simulink model "controladorContinua"  (R2021a)
settings: Solver=ode45  StartTime=0.0  StopTime=60  RelTol=1e-3
values from neighbouring files (symbols this model uses):
  AL = double(subs(A_par))    [1modeloMATEMATICOFINAL.m]    (also in modeloMATEMATICOFINAL.m)
  BL = double(subs(B_par))    [1modeloMATEMATICOFINAL.m]    (also in modeloMATEMATICOFINAL.m)
  Blo = 8.18575752786119e-06    (= 8.18575752786e-06)    [1modeloMATEMATICOFINAL.m]    (also in modeloMATEMATICOFINAL.m)
  Bmo = 2.02156082362446e-07    (= 2.02156082362e-07)    [1modeloMATEMATICOFINAL.m]    (also in modeloMATEMATICOFINAL.m)
  CL = double(subs(C_par))    [1modeloMATEMATICOFINAL.m]    (also in modeloMATEMATICOFINAL.m = [0 1 0)
  DL = double(subs(D_par))    [1modeloMATEMATICOFINAL.m]    (also in modeloMATEMATICOFINAL.m = [0)
  do = 0.06862-0.021    (= 0.04762)    [1modeloMATEMATICOFINAL.m]    (also in modeloMATEMATICOFINAL.m)
  go = 9.81    [1modeloMATEMATICOFINAL.m]    (also in modeloMATEMATICOFINAL.m)
  Jlo = 0.00100697016255642    (= 0.00100697016256)    [1modeloMATEMATICOFINAL.m]    (also in modeloMATEMATICOFINAL.m)
  Jmo = 2.08549279330578e-07    (= 2.08549279331e-07)    [1modeloMATEMATICOFINAL.m]    (also in modeloMATEMATICOFINAL.m)
  Kes = K(:,1:n)    [1modeloMATEMATICOFINAL.m]
  Ki = -K(:,n+1:end)    [1modeloMATEMATICOFINAL.m]    (also in modeloMATEMATICOFINAL.m = 3.82295123971)
  Kio = 0.00119530882984502    (= 0.00119530882985)    [1modeloMATEMATICOFINAL.m]    (also in modeloMATEMATICOFINAL.m)
  Kvo = 0.0035694528924319    (= 0.00356945289243)    [1modeloMATEMATICOFINAL.m]    (also in modeloMATEMATICOFINAL.m)
  Lo = 0.667669785204658    (= 0.667669785205)    [1modeloMATEMATICOFINAL.m]    (also in modeloMATEMATICOFINAL.m)
  mo = 0.17244    [1modeloMATEMATICOFINAL.m]    (also in modeloMATEMATICOFINAL.m)
  no = 120    [1modeloMATEMATICOFINAL.m]    (also in modeloMATEMATICOFINAL.m)
  Ro = 5.15610211779038    (= 5.15610211779)    [1modeloMATEMATICOFINAL.m]    (also in modeloMATEMATICOFINAL.m)
  Tm = 0.03    [1modeloMATEMATICOFINAL.m]    (also in modeloMATEMATICOFINAL.m)
  Vin0 = Ro*X10    (= 0)    [1modeloMATEMATICOFINAL.m]    (also in modeloMATEMATICOFINAL.m)
  X10 = 0    [1modeloMATEMATICOFINAL.m]    (also in modeloMATEMATICOFINAL.m)
  X20 = 0    [1modeloMATEMATICOFINAL.m]    (also in modeloMATEMATICOFINAL.m)
  X30 = 0    [1modeloMATEMATICOFINAL.m]    (also in modeloMATEMATICOFINAL.m)
libraries: cstblocks x12
settings Model: Creator=hubertdelgado  LastModifiedBy=hubertdelgado

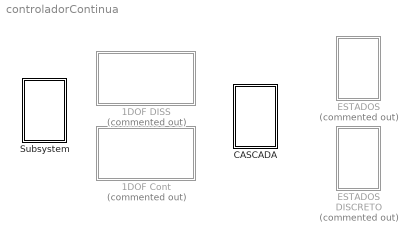
== system controladorContinua ==
  1DOF Cont : Subsystem  Commented=on
  1DOF DISS : Subsystem  Commented=on
  CASCADA : Subsystem
  ESTADOS : Subsystem  Commented=on
  ESTADOS DISCRETO : Subsystem  Commented=on
  Subsystem : Subsystem

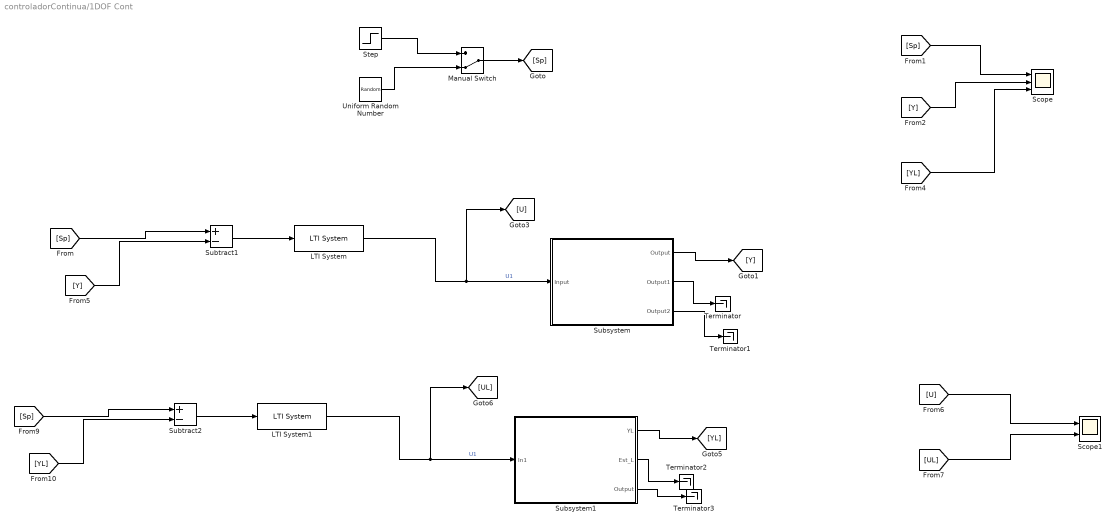
== system controladorContinua/1DOF Cont ==
  LTI System : cstblocks/LTI System  sys=Cpids  IC=[]
  LTI System1 : cstblocks/LTI System  sys=Cpids  IC=[]
  Manual Switch : ManualSwitch  CurrentSetting=0
  Scope : Scope  NumInputPorts=3
  Scope1 : Scope  NumInputPorts=2
  Step : Step  Time=0  After=0  SampleTime=0
  Subsystem : Subsystem
  Subsystem1 : Subsystem
  Subtract1 : Sum  Inputs=+-
  Subtract2 : Sum  Inputs=+-
  Terminator{,1..3} (4 alike) : Terminator
  Uniform Random Number : UniformRandomNumber  Minimum=-40*(pi/180)  Maximum=40*(pi/180)  SampleTime=8
  wires:
  Manual Switch/1 -> [Sp]
  Uniform Random Number/1 -> Manual Switch/2
  [U] -> Scope1/1
  [UL] -> Scope1/2
  Step/1 -> Manual Switch/1
  Subtract1/1 -> LTI System/1
  LTI System/1 -> Subsystem/1(Input), [U]  "U1"
  [Sp] -> Subtract1/1
  [Y] -> Subtract1/2
  Subsystem/1(Output) -> [Y]
  Subtract2/1 -> LTI System1/1
  [YL] -> Subtract2/2
  LTI System1/1 -> Subsystem1/1(In1), [UL]  "U1"
  Subsystem1/2(Est_L) -> Terminator2/1
  Subsystem1/1(YL) -> [YL]
  [Sp] -> Subtract2/1
  [Sp] -> Scope/1
  [Y] -> Scope/2
  [YL] -> Scope/3
  Subsystem/2(Output1) -> Terminator/1
  Subsystem/3(Output2) -> Terminator1/1
  Subsystem1/3(Output) -> Terminator3/1

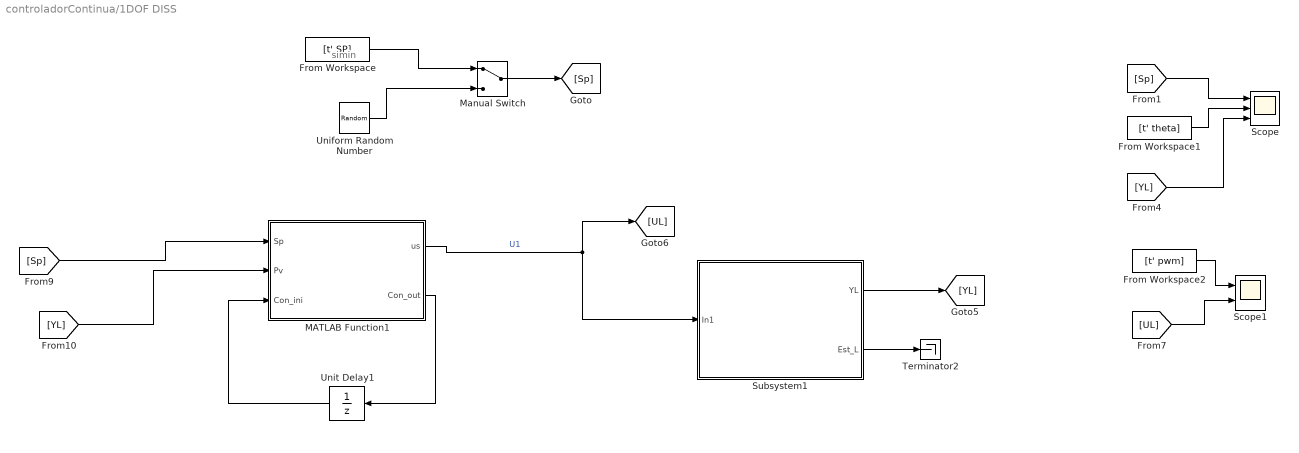
== system controladorContinua/1DOF DISS ==
  note: simin
  From Workspace : FromWorkspace  VariableName=[t' SP]
  From Workspace1 : FromWorkspace  VariableName=[t' theta]
  From Workspace2 : FromWorkspace  VariableName=[t' pwm]
  MATLAB Function1 : MATLAB Function  TreatAsAtomicUnit=on
  Manual Switch : ManualSwitch
  Scope : Scope  NumInputPorts=3
  Scope1 : Scope  NumInputPorts=2
  Subsystem1 : Subsystem
  Terminator2 : Terminator
  Uniform Random Number : UniformRandomNumber  Minimum=-40*(pi/180)  Maximum=40*(pi/180)  SampleTime=8
  Unit Delay1 : UnitDelay  InitialCondition=zeros(4,1)  SampleTime=Tm  HasFrameUpgradeWarning=on
  wires:
  Manual Switch/1 -> [Sp]
  Uniform Random Number/1 -> Manual Switch/2
  From Workspace2/1 -> Scope1/1
  [UL] -> Scope1/2
  From Workspace/1 -> Manual Switch/1
  [YL] -> MATLAB Function1/2(Pv)
  MATLAB Function1/1(us) -> Subsystem1/1(In1), [UL]  "U1"
  Subsystem1/2(Est_L) -> Terminator2/1
  Subsystem1/1(YL) -> [YL]
  [Sp] -> Scope/1
  From Workspace1/1 -> Scope/2
  [YL] -> Scope/3
  Unit Delay1/1 -> MATLAB Function1/3(Con_ini)
  [Sp] -> MATLAB Function1/1(Sp)
  MATLAB Function1/2(Con_out) -> Unit Delay1/1

== system controladorContinua/CASCADA ==
  LTI System : cstblocks/LTI System  sys=C11  IC=[]
  LTI System1 : cstblocks/LTI System  sys=G11  IC=[]
  LTI System2 : cstblocks/LTI System  sys=G21  IC=[]
  LTI System3 : cstblocks/LTI System  sys=C21  IC=[]
  MATLAB Function1 : MATLAB Function  Commented=on  TreatAsAtomicUnit=on
  Scope : Scope  NumInputPorts=2
  Scope1 : Scope  Commented=on  NumInputPorts=2
  Scope3 : Scope  Commented=on
  Subsystem1 : Subsystem  Commented=on
  Subtract : Sum  Inputs=+-
  Subtract1 : Sum  Inputs=+-
  Uniform Random Number : UniformRandomNumber  Minimum=-65*(pi/180)  Maximum=65*(pi/180)  SampleTime=8
  Unit Delay1 : UnitDelay  Commented=on  InitialCondition=zeros(8,1)  SampleTime=Tm  HasFrameUpgradeWarning=on
  wires:
  MATLAB Function1/1(u2) -> Subsystem1/1(In1), Scope3/1
  MATLAB Function1/2(Con_out) -> Unit Delay1/1
  Unit Delay1/1 -> MATLAB Function1/4(Con_ini)
  Subsystem1/1(YL) -> Scope1/2, MATLAB Function1/2(Pv)  "Pv"
  Subtract/1 -> LTI System/1  "Pv1"
  Subtract1/1 -> LTI System3/1
  LTI System2/1 -> Scope/1, Subtract1/2  "Pv"
  Uniform Random Number/1 -> Scope1/1, MATLAB Function1/1(Sp), Scope/2, Subtract1/1  "Sp"
  LTI System3/1 -> Subtract/1  "Sp1"
  LTI System/1 -> LTI System1/1
  Subsystem1/2(WL) -> MATLAB Function1/3(Pv1)
  LTI System1/1 -> Subtract/2, LTI System2/1

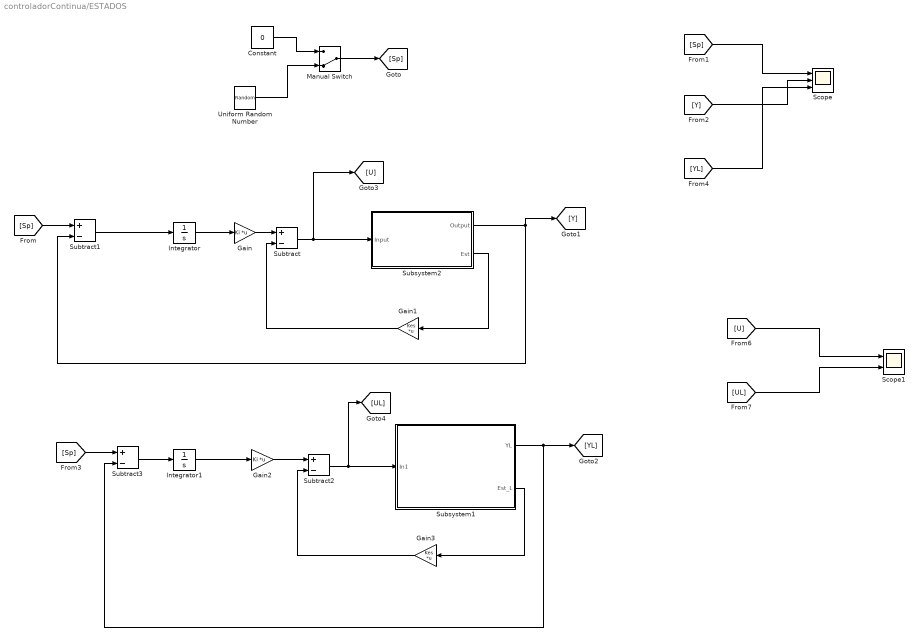
== system controladorContinua/ESTADOS ==
  Constant : Constant  Value=0
  Gain : Gain  Gain=Ki  Multiplication=Matrix(K*u)
  Gain1 : Gain  Gain=Kes  Multiplication=Matrix(K*u)
  Gain2 : Gain  Gain=Ki  Multiplication=Matrix(K*u)
  Gain3 : Gain  Gain=Kes  Multiplication=Matrix(K*u)
  Integrator : Integrator
  Integrator1 : Integrator
  Manual Switch : ManualSwitch  CurrentSetting=0
  Scope : Scope  NumInputPorts=3
  Scope1 : Scope  NumInputPorts=2
  Subsystem1 : Subsystem
  Subsystem2 : Subsystem
  Subtract{,1..3} (4 alike) : Sum  Inputs=+-
  Uniform Random Number : UniformRandomNumber  Minimum=-70*(pi/180)  Maximum=70*(pi/180)  SampleTime=8
  wires:
  Subsystem2/1(Output) -> Subtract1/2, [Y]
  Constant/1 -> Manual Switch/1
  Subsystem2/2(Est) -> Gain1/1
  Subtract/1 -> Subsystem2/1(Input), [U]
  Gain1/1 -> Subtract/2
  [YL] -> Scope/3
  Subtract2/1 -> [UL], Subsystem1/1(In1)
  Manual Switch/1 -> [Sp]
  Gain/1 -> Subtract/1
  [Sp] -> Subtract1/1
  [Sp] -> Subtract3/1
  Gain2/1 -> Subtract2/1
  Subsystem1/1(YL) -> [YL], Subtract3/2
  Subsystem1/2(Est_L) -> Gain3/1
  Gain3/1 -> Subtract2/2
  Integrator/1 -> Gain/1
  Subtract1/1 -> Integrator/1
  Integrator1/1 -> Gain2/1
  Subtract3/1 -> Integrator1/1
  Uniform Random Number/1 -> Manual Switch/2
  [Y] -> Scope/2
  [Sp] -> Scope/1
  [U] -> Scope1/1
  [UL] -> Scope1/2

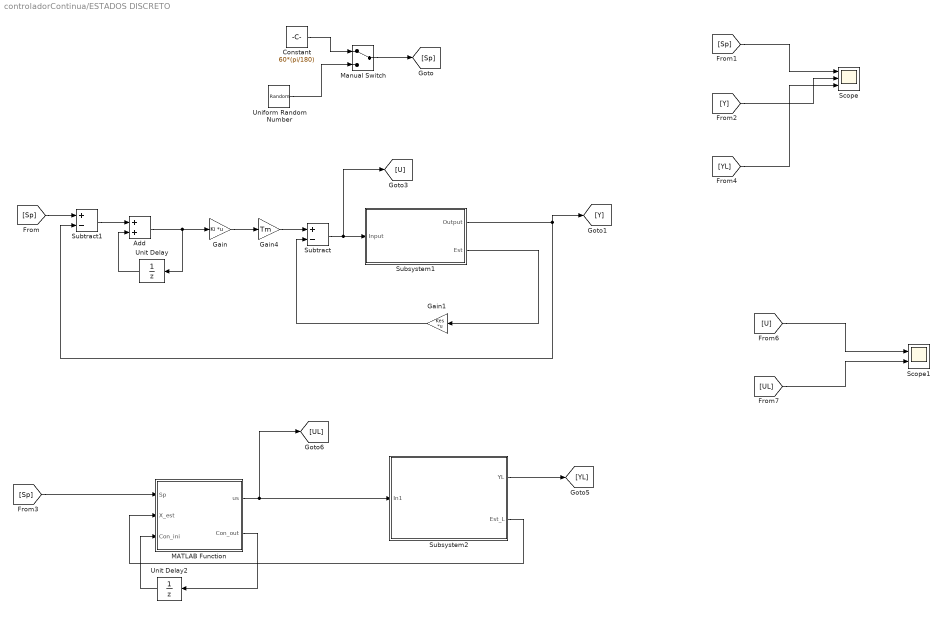
== system controladorContinua/ESTADOS DISCRETO ==
  Add : Sum
  Constant : Constant  Value=60*(pi/180)
  Gain : Gain  Gain=Ki  Multiplication=Matrix(K*u)
  Gain1 : Gain  Gain=Kes  Multiplication=Matrix(K*u)
  Gain4 : Gain  Gain=Tm
  MATLAB Function : MATLAB Function  TreatAsAtomicUnit=on
  Manual Switch : ManualSwitch
  Scope : Scope  NumInputPorts=3
  Scope1 : Scope  NumInputPorts=2
  Subsystem1 : Subsystem
  Subsystem2 : Subsystem
  Subtract : Sum  Inputs=+-
  Subtract1 : Sum  Inputs=+-
  Uniform Random Number : UniformRandomNumber  Minimum=-60*(pi/180)  Maximum=60*(pi/180)  SampleTime=8
  Unit Delay : UnitDelay  SampleTime=Tm  HasFrameUpgradeWarning=on
  Unit Delay2 : UnitDelay  InitialCondition=zeros(1,2)  SampleTime=Tm  HasFrameUpgradeWarning=on
  wires:
  Subsystem1/1(Output) -> [Y], Subtract1/2
  Subsystem1/2(Est) -> Gain1/1
  Subtract/1 -> Subsystem1/1(Input), [U]
  Gain1/1 -> Subtract/2
  [Sp] -> Subtract1/1
  Subtract1/1 -> Add/1
  Unit Delay/1 -> Add/2
  Add/1 -> Gain/1, Unit Delay/1
  Gain/1 -> Gain4/1
  Gain4/1 -> Subtract/1
  MATLAB Function/1(us) -> Subsystem2/1(In1), [UL]
  [Sp] -> MATLAB Function/1(Sp)
  MATLAB Function/2(Con_out) -> Unit Delay2/1
  Unit Delay2/1 -> MATLAB Function/3(Con_ini)
  Uniform Random Number/1 -> Manual Switch/2
  [Y] -> Scope/2
  [Sp] -> Scope/1
  [UL] -> Scope1/2
  [U] -> Scope1/1
  [YL] -> Scope/3
  Manual Switch/1 -> [Sp]
  Constant/1 -> Manual Switch/1
  Subsystem2/2(Est_L) -> MATLAB Function/2(X_est)
  Subsystem2/1(YL) -> [YL]

== system controladorContinua/Subsystem ==
  1 DOF CONTINUA : Subsystem  Commented=on
  1DOF DISCRETA : Subsystem  Commented=on
  2 DOF CONTINUA : Subsystem  Commented=on
  2 DOF DISCRETA : Subsystem  Commented=on

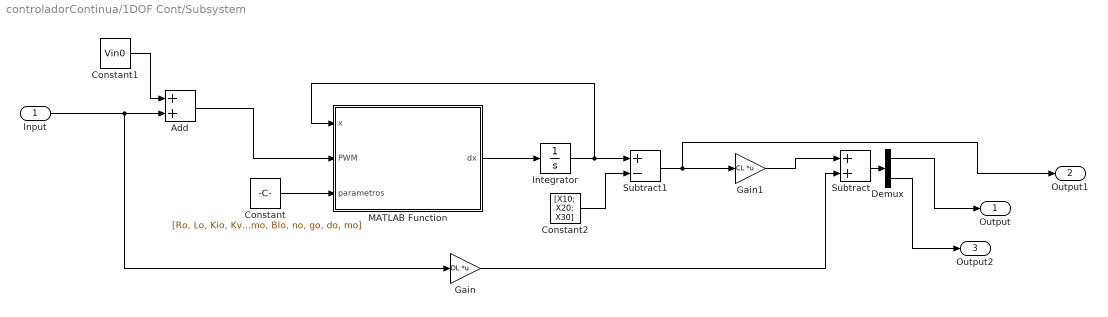
== system controladorContinua/1DOF Cont/Subsystem ==
  Input : Inport
  Add : Sum
  Constant : Constant  Value=[Ro, Lo, Kio, Kvo, Jmo, Jlo, Bmo, Blo, no, go, do, mo]
  Constant1 : Constant  Value=Vin0
  Constant2 : Constant  Value=[X10; X20; X30]
  Demux : Demux  Outputs=2
  Gain : Gain  Gain=DL  Multiplication=Matrix(K*u)
  Gain1 : Gain  Gain=CL  Multiplication=Matrix(K*u)
  Integrator : Integrator  InitialCondition=[X10; X20; X30]
  MATLAB Function : MATLAB Function  TreatAsAtomicUnit=on
  Subtract : Sum
  Subtract1 : Sum  Inputs=+-
  Output : Outport
  Output1 : Outport  Port=2
  Output2 : Outport  Port=3
  wires:
  Integrator/1 -> Subtract1/1, MATLAB Function/1(x)
  Add/1 -> MATLAB Function/2(PWM)
  Subtract1/1 -> Output1/1, Gain1/1
  MATLAB Function/1(dx) -> Integrator/1
  Constant1/1 -> Add/1
  Constant2/1 -> Subtract1/2
  Constant/1 -> MATLAB Function/3(parametros)
  Gain1/1 -> Subtract/1
  Gain/1 -> Subtract/2
  Input/1 -> Gain/1, Add/2
  Subtract/1 -> Demux/1
  Demux/1 -> Output/1
  Demux/2 -> Output2/1

== system controladorContinua/1DOF Cont/Subsystem1 ==
  In1 : Inport
  Add : Sum
  Add1 : Sum
  Demux : Demux  Outputs=2
  Gain : Gain  Gain=CL  Multiplication=Matrix(K*u)
  Gain1 : Gain  Gain=AL  Multiplication=Matrix(K*u)
  Gain2 : Gain  Gain=DL  Multiplication=Matrix(K*u)
  Gain3 : Gain  Gain=BL  Multiplication=Matrix(K*u)
  Integrator : Integrator
  YL : Outport
  Est_L : Outport  Port=2
  Output : Outport  Port=3
  wires:
  Gain/1 -> Add/2
  Integrator/1 -> Gain/1, Est_L/1, Gain1/1
  Add1/1 -> Integrator/1
  Gain1/1 -> Add1/2
  Gain2/1 -> Add/1
  Gain3/1 -> Add1/1
  In1/1 -> Gain2/1, Gain3/1
  Add/1 -> Demux/1
  Demux/1 -> YL/1
  Demux/2 -> Output/1

== system controladorContinua/1DOF DISS/Subsystem1 ==
  In1 : Inport
  Add : Sum
  Add1 : Sum
  Gain : Gain  Gain=CL  Multiplication=Matrix(K*u)
  Gain1 : Gain  Gain=AL  Multiplication=Matrix(K*u)
  Gain2 : Gain  Gain=DL  Multiplication=Matrix(K*u)
  Gain3 : Gain  Gain=BL  Multiplication=Matrix(K*u)
  Integrator : Integrator
  YL : Outport
  Est_L : Outport  Port=2
  wires:
  Gain/1 -> Add/2
  Integrator/1 -> Gain/1, Est_L/1, Gain1/1
  Add1/1 -> Integrator/1
  Gain1/1 -> Add1/2
  Gain2/1 -> Add/1
  Gain3/1 -> Add1/1
  Add/1 -> YL/1
  In1/1 -> Gain2/1, Gain3/1

== system controladorContinua/CASCADA/Subsystem1 ==
  In1 : Inport
  Add : Sum
  Add1 : Sum
  Demux : Demux  Outputs=2
  Gain : Gain  Gain=CL  Multiplication=Matrix(K*u)
  Gain1 : Gain  Gain=AL  Multiplication=Matrix(K*u)
  Gain2 : Gain  Gain=DL  Multiplication=Matrix(K*u)
  Gain3 : Gain  Gain=BL  Multiplication=Matrix(K*u)
  Integrator : Integrator
  YL : Outport
  WL : Outport  Port=2
  wires:
  Gain/1 -> Add/2
  Integrator/1 -> Gain/1, Gain1/1
  Add1/1 -> Integrator/1
  Gain1/1 -> Add1/2
  Gain2/1 -> Add/1
  Gain3/1 -> Add1/1
  In1/1 -> Gain2/1, Gain3/1
  Add/1 -> Demux/1
  Demux/1 -> YL/1
  Demux/2 -> WL/1

== system controladorContinua/ESTADOS/Subsystem1 ==
  In1 : Inport
  Add : Sum
  Add1 : Sum
  Gain : Gain  Gain=CL  Multiplication=Matrix(K*u)
  Gain1 : Gain  Gain=AL  Multiplication=Matrix(K*u)
  Gain2 : Gain  Gain=DL  Multiplication=Matrix(K*u)
  Gain3 : Gain  Gain=BL  Multiplication=Matrix(K*u)
  Integrator : Integrator
  YL : Outport
  Est_L : Outport  Port=2
  wires:
  Gain/1 -> Add/2
  Integrator/1 -> Gain/1, Est_L/1, Gain1/1
  Add1/1 -> Integrator/1
  Gain1/1 -> Add1/2
  Gain2/1 -> Add/1
  Gain3/1 -> Add1/1
  Add/1 -> YL/1
  In1/1 -> Gain2/1, Gain3/1

== system controladorContinua/ESTADOS/Subsystem2 ==
  Input : Inport
  Add : Sum
  Constant : Constant  Value=[Ro,Lo,Kio, Kvo, Jmo, Jlo, Bmo, Blo, no, go, do, mo]
  Constant1 : Constant  Value=Vin0
  Constant2 : Constant  Value=[X10; X20]
  Gain1 : Gain  Gain=CL  Multiplication=Matrix(K*u)
  Integrator : Integrator  InitialCondition=[X10; X20]
  MATLAB Function : MATLAB Function  TreatAsAtomicUnit=on
  Subtract1 : Sum  Inputs=+-
  Output : Outport
  Est : Outport  Port=2
  wires:
  Add/1 -> MATLAB Function/2(PWM)
  Constant2/1 -> Subtract1/2
  Constant1/1 -> Add/1
  Input/1 -> Add/2
  MATLAB Function/1(dx) -> Integrator/1
  Constant/1 -> MATLAB Function/3(parametros)
  Integrator/1 -> Subtract1/1, MATLAB Function/1(x)
  Subtract1/1 -> Est/1, Gain1/1
  Gain1/1 -> Output/1

== system controladorContinua/ESTADOS DISCRETO/Subsystem1 ==
  Input : Inport
  Add : Sum
  Constant : Constant  Value=[Ro,Lo,Kio, Kvo, Jmo, Jlo, Bmo, Blo, no, go, do, mo]
  Constant1 : Constant  Value=Vin0
  Constant2 : Constant  Value=[X10; X20]
  Gain1 : Gain  Gain=CL  Multiplication=Matrix(K*u)
  Integrator : Integrator  InitialCondition=[X10; X20]
  MATLAB Function : MATLAB Function  TreatAsAtomicUnit=on
  Subtract1 : Sum  Inputs=+-
  Output : Outport
  Est : Outport  Port=2
  wires:
  Add/1 -> MATLAB Function/2(PWM)
  Constant2/1 -> Subtract1/2
  Constant1/1 -> Add/1
  Input/1 -> Add/2
  MATLAB Function/1(dx) -> Integrator/1
  Constant/1 -> MATLAB Function/3(parametros)
  Integrator/1 -> Subtract1/1, MATLAB Function/1(x)
  Subtract1/1 -> Est/1, Gain1/1
  Gain1/1 -> Output/1

== system controladorContinua/ESTADOS DISCRETO/Subsystem2 ==
  In1 : Inport
  Add : Sum
  Add1 : Sum
  Gain : Gain  Gain=CL  Multiplication=Matrix(K*u)
  Gain1 : Gain  Gain=AL  Multiplication=Matrix(K*u)
  Gain2 : Gain  Gain=DL  Multiplication=Matrix(K*u)
  Gain3 : Gain  Gain=BL  Multiplication=Matrix(K*u)
  Integrator : Integrator
  YL : Outport
  Est_L : Outport  Port=2
  wires:
  Gain/1 -> Add/2
  Integrator/1 -> Gain/1, Est_L/1, Gain1/1
  Add1/1 -> Integrator/1
  Gain1/1 -> Add1/2
  Gain2/1 -> Add/1
  Gain3/1 -> Add1/1
  Add/1 -> YL/1
  In1/1 -> Gain2/1, Gain3/1

== system controladorContinua/Subsystem/1 DOF CONTINUA ==
  Demux : Demux  Outputs=1
  LTI System : cstblocks/LTI System  sys=Cpids  IC=[]
  LTI System1 : cstblocks/LTI System  sys=Cpids  IC=[]
  Scope : Scope  NumInputPorts=3
  Scope1 : Scope
  Scope3 : Scope
  Scope4 : Scope  NumInputPorts=2
  State-Space : StateSpace  A=AL  B=BL  C=CL  D=DL  InitialCondition=[0;0;0]
  Subsystem : Subsystem
  Subtract : Sum  Inputs=+-
  Subtract1 : Sum  Inputs=+-
  Uniform Random Number : UniformRandomNumber  Minimum=-65*(pi/180)  Maximum=65*(pi/180)  SampleTime=8
  wires:
  LTI System/1 -> Scope4/1, State-Space/1  "U4"
  Subsystem/2(Output1) -> Scope3/1
  Subtract1/1 -> LTI System1/1  "E1"
  Subtract/1 -> LTI System/1  "E1"
  LTI System1/1 -> Scope4/2, Subsystem/1(Input)  "U4"
  Subsystem/1(Output) -> Scope/3, Subtract1/2
  State-Space/1 -> Demux/1
  Uniform Random Number/1 -> Subtract/1, Scope/1, Subtract1/1
  Demux/1 -> Scope/2, Subtract/2
  ? -> Scope1/1

== system controladorContinua/Subsystem/1DOF DISCRETA ==
  Demux : Demux  Outputs=2
  MATLAB Function : MATLAB Function  TreatAsAtomicUnit=on
  MATLAB Function1 : MATLAB Function  TreatAsAtomicUnit=on
  Scope : Scope  NumInputPorts=3
  Scope2 : Scope
  Scope3 : Scope
  Scope4 : Scope  NumInputPorts=2
  State-Space1 : StateSpace  A=AL  B=BL  C=CL  D=DL  InitialCondition=[0;0;0]
  Subsystem : Subsystem
  Uniform Random Number : UniformRandomNumber  Minimum=-65*(pi/180)  Maximum=65*(pi/180)  SampleTime=8
  Unit Delay : UnitDelay  InitialCondition=zeros(4,1)  SampleTime=Tm  HasFrameUpgradeWarning=on
  Unit Delay1 : UnitDelay  InitialCondition=zeros(4,1)  SampleTime=Tm  HasFrameUpgradeWarning=on
  wires:
  Subsystem/2(Output1) -> Scope3/1
  MATLAB Function1/1(us) -> Subsystem/1(Input)  "U4"
  MATLAB Function/1(us) -> Scope4/1, State-Space1/1  "Cod"
  Demux/2 -> Scope2/1
  Unit Delay/1 -> MATLAB Function/3(Con_ini)
  State-Space1/1 -> Demux/1
  MATLAB Function1/2(Con_out) -> Unit Delay1/1
  Demux/1 -> MATLAB Function/2(Pv), Scope/2
  Uniform Random Number/1 -> Scope/1, MATLAB Function/1(Sp), MATLAB Function1/1(Sp)
  Unit Delay1/1 -> MATLAB Function1/3(Con_ini)
  Subsystem/1(Output) -> MATLAB Function1/2(Pv)
  MATLAB Function/2(Con_out) -> Unit Delay/1
  ? -> Scope/3
  ? -> Scope4/2

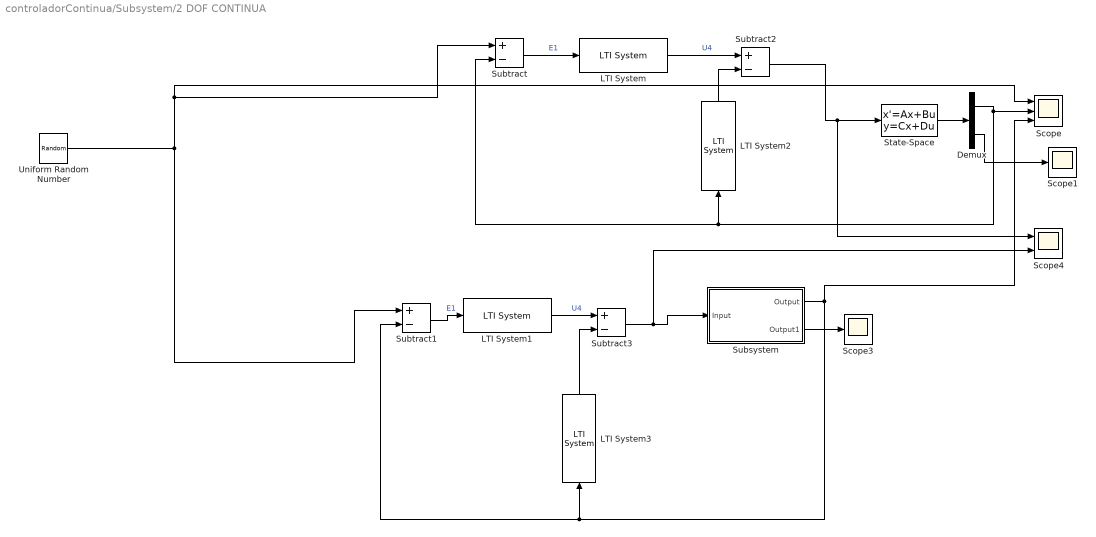
== system controladorContinua/Subsystem/2 DOF CONTINUA ==
  Demux : Demux  Outputs=2
  LTI System : cstblocks/LTI System  sys=C1s  IC=[]
  LTI System1 : cstblocks/LTI System  sys=C1s  IC=[]
  LTI System2 : cstblocks/LTI System  sys=C2s  IC=[]
  LTI System3 : cstblocks/LTI System  sys=C2s  IC=[]
  Scope : Scope  NumInputPorts=3
  Scope1 : Scope
  Scope3 : Scope
  Scope4 : Scope  NumInputPorts=2
  State-Space : StateSpace  A=AL  B=BL  C=CL  D=DL  InitialCondition=[0;0;0]
  Subsystem : Subsystem
  Subtract{,1..3} (4 alike) : Sum  Inputs=+-
  Uniform Random Number : UniformRandomNumber  Minimum=-40*(pi/180)  Maximum=40*(pi/180)  SampleTime=8
  wires:
  Subsystem/2(Output1) -> Scope3/1
  Subtract1/1 -> LTI System1/1  "E1"
  Subtract/1 -> LTI System/1  "E1"
  Subsystem/1(Output) -> Scope/3, LTI System3/1, Subtract1/2
  State-Space/1 -> Demux/1
  Uniform Random Number/1 -> Subtract/1, Scope/1, Subtract1/1
  Demux/1 -> LTI System2/1, Subtract/2, Scope/2
  Demux/2 -> Scope1/1
  LTI System/1 -> Subtract2/1  "U4"
  Subtract2/1 -> Scope4/1, State-Space/1
  LTI System2/1 -> Subtract2/2
  LTI System1/1 -> Subtract3/1  "U4"
  Subtract3/1 -> Scope4/2, Subsystem/1(Input)
  LTI System3/1 -> Subtract3/2

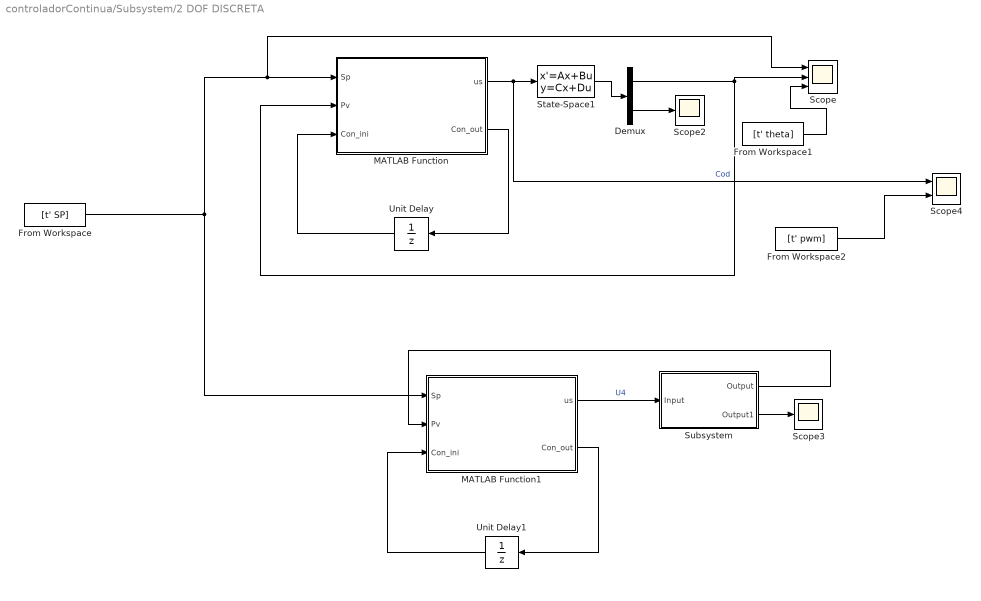
== system controladorContinua/Subsystem/2 DOF DISCRETA ==
  Demux : Demux  Outputs=2
  From Workspace : FromWorkspace  VariableName=[t' SP]
  From Workspace1 : FromWorkspace  VariableName=[t' theta]
  From Workspace2 : FromWorkspace  VariableName=[t' pwm]
  MATLAB Function : MATLAB Function  TreatAsAtomicUnit=on
  MATLAB Function1 : MATLAB Function  TreatAsAtomicUnit=on
  Scope : Scope  NumInputPorts=3
  Scope2 : Scope
  Scope3 : Scope
  Scope4 : Scope  NumInputPorts=2
  State-Space1 : StateSpace  A=AL  B=BL  C=CL  D=DL  InitialCondition=[0;0;0]
  Subsystem : Subsystem
  Unit Delay : UnitDelay  InitialCondition=zeros(6,1)  SampleTime=Tm  HasFrameUpgradeWarning=on
  Unit Delay1 : UnitDelay  InitialCondition=zeros(6,1)  SampleTime=Tm  HasFrameUpgradeWarning=on
  wires:
  Subsystem/2(Output1) -> Scope3/1
  MATLAB Function1/1(us) -> Subsystem/1(Input)  "U4"
  MATLAB Function/1(us) -> Scope4/1, State-Space1/1  "Cod"
  Demux/2 -> Scope2/1
  Unit Delay/1 -> MATLAB Function/3(Con_ini)
  State-Space1/1 -> Demux/1
  MATLAB Function1/2(Con_out) -> Unit Delay1/1
  Demux/1 -> MATLAB Function/2(Pv), Scope/2
  From Workspace/1 -> MATLAB Function1/1(Sp), Scope/1, MATLAB Function/1(Sp)
  Unit Delay1/1 -> MATLAB Function1/3(Con_ini)
  MATLAB Function/2(Con_out) -> Unit Delay/1
  Subsystem/1(Output) -> MATLAB Function1/2(Pv)
  From Workspace2/1 -> Scope4/2
  From Workspace1/1 -> Scope/3

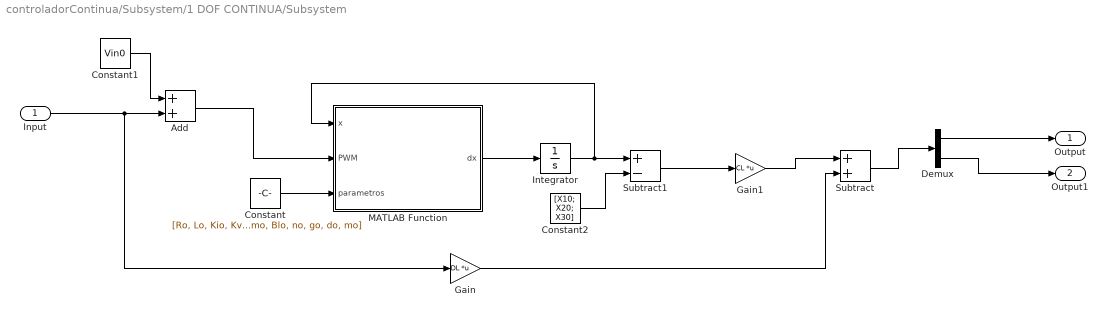
== system controladorContinua/Subsystem/1 DOF CONTINUA/Subsystem ==
  Input : Inport
  Add : Sum
  Constant : Constant  Value=[Ro, Lo, Kio, Kvo, Jmo, Jlo, Bmo, Blo, no, go, do, mo]
  Constant1 : Constant  Value=Vin0
  Constant2 : Constant  Value=[X10; X20; X30]
  Demux : Demux  Outputs=2
  Gain : Gain  Gain=DL  Multiplication=Matrix(K*u)
  Gain1 : Gain  Gain=CL  Multiplication=Matrix(K*u)
  Integrator : Integrator  InitialCondition=[X10; X20; X30]
  MATLAB Function : MATLAB Function  TreatAsAtomicUnit=on
  Subtract : Sum
  Subtract1 : Sum  Inputs=+-
  Output : Outport
  Output1 : Outport  Port=2
  wires:
  Subtract/1 -> Demux/1
  Gain1/1 -> Subtract/1
  Demux/2 -> Output1/1
  Subtract1/1 -> Gain1/1
  Integrator/1 -> Subtract1/1, MATLAB Function/1(x)
  Constant/1 -> MATLAB Function/3(parametros)
  MATLAB Function/1(dx) -> Integrator/1
  Demux/1 -> Output/1
  Constant1/1 -> Add/1
  Gain/1 -> Subtract/2
  Constant2/1 -> Subtract1/2
  Add/1 -> MATLAB Function/2(PWM)
  Input/1 -> Gain/1, Add/2

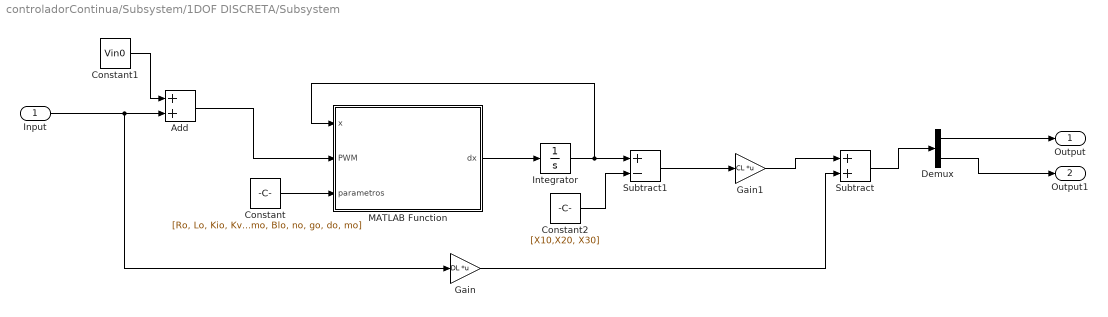
== system controladorContinua/Subsystem/1DOF DISCRETA/Subsystem ==
  Input : Inport
  Add : Sum
  Constant : Constant  Value=[Ro, Lo, Kio, Kvo, Jmo, Jlo, Bmo, Blo, no, go, do, mo]
  Constant1 : Constant  Value=Vin0
  Constant2 : Constant  Value=[X10,X20, X30]
  Demux : Demux  Outputs=2
  Gain : Gain  Gain=DL  Multiplication=Matrix(K*u)
  Gain1 : Gain  Gain=CL  Multiplication=Matrix(K*u)
  Integrator : Integrator  InitialCondition=[X10; X20; X30]
  MATLAB Function : MATLAB Function  TreatAsAtomicUnit=on
  Subtract : Sum
  Subtract1 : Sum  Inputs=+-
  Output : Outport
  Output1 : Outport  Port=2
  wires:
  Subtract/1 -> Demux/1
  Gain1/1 -> Subtract/1
  Demux/2 -> Output1/1
  Subtract1/1 -> Gain1/1
  Integrator/1 -> Subtract1/1, MATLAB Function/1(x)
  Constant/1 -> MATLAB Function/3(parametros)
  MATLAB Function/1(dx) -> Integrator/1
  Demux/1 -> Output/1
  Constant1/1 -> Add/1
  Gain/1 -> Subtract/2
  Constant2/1 -> Subtract1/2
  Add/1 -> MATLAB Function/2(PWM)
  Input/1 -> Gain/1, Add/2

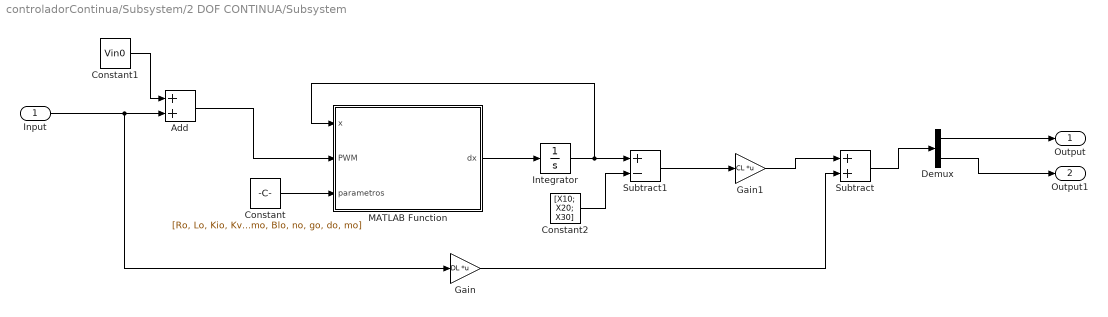
== system controladorContinua/Subsystem/2 DOF CONTINUA/Subsystem ==
  Input : Inport
  Add : Sum
  Constant : Constant  Value=[Ro, Lo, Kio, Kvo, Jmo, Jlo, Bmo, Blo, no, go, do, mo]
  Constant1 : Constant  Value=Vin0
  Constant2 : Constant  Value=[X10; X20; X30]
  Demux : Demux  Outputs=2
  Gain : Gain  Gain=DL  Multiplication=Matrix(K*u)
  Gain1 : Gain  Gain=CL  Multiplication=Matrix(K*u)
  Integrator : Integrator  InitialCondition=[X10; X20; X30]
  MATLAB Function : MATLAB Function  TreatAsAtomicUnit=on
  Subtract : Sum
  Subtract1 : Sum  Inputs=+-
  Output : Outport
  Output1 : Outport  Port=2
  wires:
  Subtract/1 -> Demux/1
  Gain1/1 -> Subtract/1
  Demux/2 -> Output1/1
  Subtract1/1 -> Gain1/1
  Integrator/1 -> Subtract1/1, MATLAB Function/1(x)
  Constant/1 -> MATLAB Function/3(parametros)
  MATLAB Function/1(dx) -> Integrator/1
  Demux/1 -> Output/1
  Constant1/1 -> Add/1
  Gain/1 -> Subtract/2
  Constant2/1 -> Subtract1/2
  Add/1 -> MATLAB Function/2(PWM)
  Input/1 -> Gain/1, Add/2

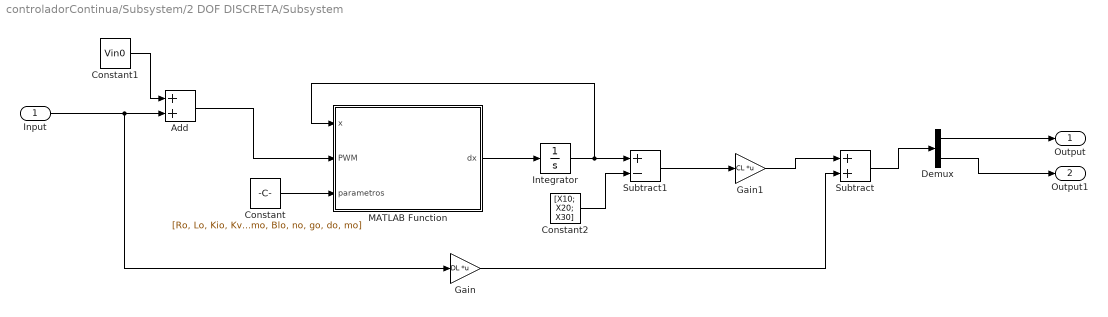
== system controladorContinua/Subsystem/2 DOF DISCRETA/Subsystem ==
  Input : Inport
  Add : Sum
  Constant : Constant  Value=[Ro, Lo, Kio, Kvo, Jmo, Jlo, Bmo, Blo, no, go, do, mo]
  Constant1 : Constant  Value=Vin0
  Constant2 : Constant  Value=[X10; X20; X30]
  Demux : Demux  Outputs=2
  Gain : Gain  Gain=DL  Multiplication=Matrix(K*u)
  Gain1 : Gain  Gain=CL  Multiplication=Matrix(K*u)
  Integrator : Integrator  InitialCondition=[X10; X20; X30]
  MATLAB Function : MATLAB Function  TreatAsAtomicUnit=on
  Subtract : Sum
  Subtract1 : Sum  Inputs=+-
  Output : Outport
  Output1 : Outport  Port=2
  wires:
  Subtract/1 -> Demux/1
  Gain1/1 -> Subtract/1
  Demux/2 -> Output1/1
  Subtract1/1 -> Gain1/1
  Integrator/1 -> Subtract1/1, MATLAB Function/1(x)
  Constant/1 -> MATLAB Function/3(parametros)
  MATLAB Function/1(dx) -> Integrator/1
  Demux/1 -> Output/1
  Constant1/1 -> Add/1
  Gain/1 -> Subtract/2
  Constant2/1 -> Subtract1/2
  Add/1 -> MATLAB Function/2(PWM)
  Input/1 -> Gain/1, Add/2

== matlab function controladorContinua/ESTADOS DISCRETO/Subsystem1/MATLAB Function ==
  data: x input; PWM input; dx output; parametros input
function dx = fcn(x,PWM,parametros)

%ESTADOS
x1 = x(1);
x2 = x(2);

%Parametros
R = parametros(1);
L = parametros(2);
Ki = parametros(3);
Kv = parametros(4);
Jm = parametros(5);
Jl = parametros(6);
Bm = parametros(7);
Bl = parametros(8);
n = parametros(9);
g = parametros(10);
d = parametros(11);
m = parametros(12);

%EXPRESIONES
f1 = x2; %d0l/dt = Wl
f2= ((Ki*(((7*PWM/100)-(Kv*x2*n)/R))*n)-x2*(Bm*n^2+Bl)-(m*g*d*sin(x1)))/(Jl+Jm*n^2);

dx = [f1; f2];

== matlab function controladorContinua/Subsystem/1DOF DISCRETA/Subsystem/MATLAB Function ==
  data: x input; PWM input; dx output; parametros input
function dx = fcn(x,PWM,parametros)

%ESTADOS
x1 = x(1);
x2 = x(2);
x3 = x(3);

%Parametros
R = parametros(1);
L = parametros(2);
Ki = parametros(3);
Kv = parametros(4);
Jm = parametros(5);
Jl = parametros(6);
Bm = parametros(7);
Bl = parametros(8);
n = parametros(9);
g = parametros(10);
d = parametros(11);
m = parametros(12);

%EXPRESIONES
% Jt = Jm*n^2 +Jl;
% f1 = (1/L)*(((7*PWM)/100) - R*x1 - Kv*x2*n);
% f2 = (1/Jt)*(Ki*x1*n - (Bm*n^2 + Bl)*x2 - m*g*d*sin(x3));
% f3 = x2;

% MODELO 2 ESTADOS I TL WL  SALIDA TL WL
f1 = (((7*PWM)/100)-Kv*x3*n-R*x1)/(L); %di/dt
f2 = x3; %d0l/dt = Wl
f3 = ((Ki*x1*n)-x3*(Bm*n^2+Bl)-(m*g*d*sin(x2)))/(Jl+Jm*n^2);  %dwl/dt 

dx = [f1; f2; f3];

== matlab function controladorContinua/1DOF Cont/Subsystem/MATLAB Function ==
  data: x input; PWM input; dx output; parametros input
function dx = fcn(x,PWM,parametros)

%ESTADOS
x1 = x(1);
x2 = x(2);
x3 = x(3);

%Parametros
R = parametros(1);
L = parametros(2);
Ki = parametros(3);
Kv = parametros(4);
Jm = parametros(5);
Jl = parametros(6);
Bm = parametros(7);
Bl = parametros(8);
n = parametros(9);
g = parametros(10);
d = parametros(11);
m = parametros(12);

%EXPRESIONES
% Jt = Jm*n^2 +Jl;
% f1 = (1/L)*(((7*PWM)/100) - R*x1 - Kv*x2*n);
% f2 = (1/Jt)*(Ki*x1*n - (Bm*n^2 + Bl)*x2 - m*g*d*sin(x3));
% f3 = x2;

% MODELO 2 ESTADOS I TL WL  SALIDA TL WL
f1 = (((7*PWM)/100)-Kv*x3*n-R*x1)/(L); %di/dt
f2 = x3; %d0l/dt = Wl
f3 = ((Ki*x1*n)-x3*(Bm*n^2+Bl)-(m*g*d*sin(x2)))/(Jl+Jm*n^2);  %dwl/dt 

dx = [f1; f2; f3];

== matlab function controladorContinua/ESTADOS DISCRETO/MATLAB Function ==
  data: Sp input; us output; X_est input; Con_ini input; Con_out output
function [us,Con_out] = fcn(Sp,X_est,Con_ini)

umax = 100;
umin = -100;
kaw = zeros(1);
CL = [1, 0]
Ki = [13.038404810405284];
Kes = [8.39272964861829,6.19627625077861];

Vk_1 = Con_ini(1);
dif_act = Con_ini(2);

Tm = 0.03;
Kid = Ki*Tm;

Pv = CL*X_est;
en = Sp - Pv;
Vk = en + Vk_1 + kaw*dif_act;
un = Kid*Vk - Kes*X_est;
us = un;

Vk_1 = Vk;

if un>umax
    us = umax;
end
if un<umin
    us = umin;
end

dif_act = us - un;
Con_out = [Vk_1; dif_act];

== matlab function controladorContinua/1DOF DISS/MATLAB Function1 ==
  data: Sp input; us output; Pv input; Con_ini input; Con_out output
% function [us, Con_out] = fcn(Sp, Pv, Con_ini)
%  
% en_1 = Con_ini(1);
% en_2 = Con_ini(2);
% un_1 = Con_ini(3);
% un_2 = Con_ini(4);
% difact = Con_ini(5);
% umin = -100;
% umax = 100;
% kaw = 0.1; 
%  
% en = Sp - Pv;
% un = 52.346730287862997*en - 99.613623826288730*en_1 + 48.365148241217845*en_2 + 1.742509213223832*un_1 - 0.742509213223832*un_2 + kaw*difact;
%  
% us = un;
%  
% if un < umin 
%     us = umin;
% end
% if un > umax 
%     us = umax;
% end
%  
% en_2 = en_1;
% en_1 = en;
% un_2 = un_1;
% un_1 = un;
% difact = us - un;
%          
% Con_out = [en_1; en_2; un_1; un_2; difact];

function [us, Con_out] = fcn(Sp, Pv, Con_ini)

en_1 = Con_ini(1);
I_error_1 = Con_ini(2);
difact = Con_ini(3);
Ad_1 = Con_ini(4);

umin = -100;
umax = 100;

Kp = -1.101543753570772;
Ki = 2.065219414420463
Kd = 30.183054627013306;
N = 0.742509213223832;
kaw=0.1; 


en = Sp - Pv;
Ap = Kp*en;
Ad = Kd*(en-en_1) + N*Ad_1;
I_error = en + I_error_1 + kaw*difact;
Ai = Ki*I_error;
un = Ap + Ai + Ad;
us = un;

if un < umin 
    us = umin;
end
if un > umax 
    us = umax;
end

en_1 = en;
I_error_1 = I_error;
difact = us - un;
Ad_1 = Ad;
      
Con_out = [en_1; I_error_1; difact; Ad_1];

== matlab function controladorContinua/Subsystem/1 DOF CONTINUA/Subsystem/MATLAB Function ==
  data: x input; PWM input; dx output; parametros input
function dx = fcn(x,PWM,parametros)

%ESTADOS
x1 = x(1);
x2 = x(2);
x3 = x(3);

%Parametros
R = parametros(1);
L = parametros(2);
Ki = parametros(3);
Kv = parametros(4);
Jm = parametros(5);
Jl = parametros(6);
Bm = parametros(7);
Bl = parametros(8);
n = parametros(9);
g = parametros(10);
d = parametros(11);
m = parametros(12);

%EXPRESIONES
% Jt = Jm*n^2 +Jl;
% f1 = (1/L)*(((7*PWM)/100) - R*x1 - Kv*x2*n);
% f2 = (1/Jt)*(Ki*x1*n - (Bm*n^2 + Bl)*x2 - m*g*d*sin(x3));
% f3 = x2;

% MODELO 2 ESTADOS I TL WL  SALIDA TL WL
f1 = (((7*PWM)/100)-Kv*x3*n-R*x1)/(L); %di/dt
f2 = x3; %d0l/dt = Wl
f3 = ((Ki*x1*n)-x3*(Bm*n^2+Bl)-(m*g*d*sin(x2)))/(Jl+Jm*n^2);  %dwl/dt 

dx = [f1; f2; f3];

== matlab function controladorContinua/Subsystem/1DOF DISCRETA/MATLAB Function1 ==
  data: Sp input; us output; Pv input; Con_ini input; Con_out output
% function [us, Con_out] = fcn(Sp, Pv, Con_ini)
%  
% en_1 = Con_ini(1);
% en_2 = Con_ini(2);
% un_1 = Con_ini(3);
% un_2 = Con_ini(4);
% difact = Con_ini(5);
% umin = -100;
% umax = 100;
% kaw = 0.1; 
%  
% en = Sp - Pv;
% un = 52.346730287862997*en - 99.613623826288730*en_1 + 48.365148241217845*en_2 + 1.742509213223832*un_1 - 0.742509213223832*un_2 + kaw*difact;
%  
% us = un;
%  
% if un < umin 
%     us = umin;
% end
% if un > umax 
%     us = umax;
% end
%  
% en_2 = en_1;
% en_1 = en;
% un_2 = un_1;
% un_1 = un;
% difact = us - un;
%          
% Con_out = [en_1; en_2; un_1; un_2; difact];

function [us, Con_out] = fcn(Sp, Pv, Con_ini)

en_1 = Con_ini(1);
I_error_1 = Con_ini(2);
difact = Con_ini(3);
Ad_1 = Con_ini(4);

umin = -100;
umax = 100;

Kp = -1.101543753570772;
Ki = 4.265219414420463;
Kd = 49.183054627013306;
N = 0.742509213223832;
kaw=0.1; 


en = Sp - Pv;
Ap = Kp*en;
Ad = Kd*(en-en_1) + N*Ad_1;
I_error = en + I_error_1 + kaw*difact;
Ai = Ki*I_error;
un = Ap + Ai + Ad;
us = un;

if un < umin 
    us = umin;
end
if un > umax 
    us = umax;
end

en_1 = en;
I_error_1 = I_error;
difact = us - un;
Ad_1 = Ad;
      
Con_out = [en_1; I_error_1; difact; Ad_1];

== matlab function controladorContinua/Subsystem/2 DOF CONTINUA/Subsystem/MATLAB Function ==
  data: x input; PWM input; dx output; parametros input
function dx = fcn(x,PWM,parametros)

%ESTADOS
x1 = x(1);
x2 = x(2);
x3 = x(3);

%Parametros
R = parametros(1);
L = parametros(2);
Ki = parametros(3);
Kv = parametros(4);
Jm = parametros(5);
Jl = parametros(6);
Bm = parametros(7);
Bl = parametros(8);
n = parametros(9);
g = parametros(10);
d = parametros(11);
m = parametros(12);

%EXPRESIONES
% Jt = Jm*n^2 +Jl;
% f1 = (1/L)*(((7*PWM)/100) - R*x1 - Kv*x2*n);
% f2 = (1/Jt)*(Ki*x1*n - (Bm*n^2 + Bl)*x2 - m*g*d*sin(x3));
% f3 = x2;

% MODELO 2 ESTADOS I TL WL  SALIDA TL WL
f1 = (((7*PWM)/100)-Kv*x3*n-R*x1)/(L); %di/dt
f2 = x3; %d0l/dt = Wl
f3 = ((Ki*x1*n)-x3*(Bm*n^2+Bl)-(m*g*d*sin(x2)))/(Jl+Jm*n^2);  %dwl/dt 

dx = [f1; f2; f3];

== matlab function controladorContinua/Subsystem/1DOF DISCRETA/MATLAB Function ==
  data: Sp input; us output; Pv input; Con_ini input; Con_out output
% function [us, Con_out] = fcn(Sp, Pv, Con_ini)
%  
% en_1 = Con_ini(1);
% en_2 = Con_ini(2);
% un_1 = Con_ini(3);
% un_2 = Con_ini(4);
% difact = Con_ini(5);
% umin = -100;
% umax = 100;
% kaw = 0.1; 
%  
% en = Sp - Pv;
% un = 52.346730287862997*en - 99.613623826288730*en_1 + 48.365148241217845*en_2 + 1.742509213223832*un_1 - 0.742509213223832*un_2 + kaw*difact;
%  
% us = un;
%  
% if un < umin 
%     us = umin;
% end
% if un > umax 
%     us = umax;
% end
%  
% en_2 = en_1;
% en_1 = en;
% un_2 = un_1;
% un_1 = un;
% difact = us - un;
%          
% Con_out = [en_1; en_2; un_1; un_2; difact];

function [us, Con_out] = fcn(Sp, Pv, Con_ini)

en_1 = Con_ini(1);
I_error_1 = Con_ini(2);
difact = Con_ini(3);
Ad_1 = Con_ini(4);

umin = -100;
umax = 100;

Kp = -1.101543753570772;
Ki = 4.265219414420463;
Kd = 49.183054627013306;
N = 0.742509213223832;
kaw=0.1; 


en = Sp - Pv;
Ap = Kp*en;
Ad = Kd*(en-en_1) + N*Ad_1;
I_error = en + I_error_1 + kaw*difact;
Ai = Ki*I_error;
un = Ap + Ai + Ad;
us = un;

if un < umin 
    us = umin;
end
if un > umax 
    us = umax;
end

en_1 = en;
I_error_1 = I_error;
difact = us - un;
Ad_1 = Ad;
      
Con_out = [en_1; I_error_1; difact; Ad_1];

== matlab function controladorContinua/Subsystem/2 DOF DISCRETA/MATLAB Function ==
  data: Sp input; us output; Pv input; Con_ini input; Con_out output
% function [us, Con_out] = fcn(Sp, Pv, Con_ini)
%  
% en_1 = Con_ini(1);
% u1_1 = Con_ini(2);
% Pv_1 = Con_ini(3);
% u2_1 = Con_ini(4);
% difact = Con_ini(5);
% umin = -100;
% umax = 100;
% kaw = 0.01; 
%  
% en = Sp - Pv;
% u1 = 0.153958966653420*en_1 + u1_1 + kaw*difact;
% u2 = 22.177058343736231*Pv - 21.573923642220816*(Pv_1) + 0.732201155629244*u2_1;
% un = u1-u2;
% us = un;
%  
% if un < umin 
%     us = umin;
% end
% if un > umax 
%     us = umax;
% end
%  
% en_1 = en;
% u1_1 = u1;
% Pv_1 = Pv;
% u2_1 = u2;
% difact = us - un;
%          
% Con_out = [en_1; u1_1; Pv_1;u2_1; difact];

function [us, Con_out] = fcn(Sp, Pv, Con_ini)

en_1 = Con_ini(1);
yn_1 = Con_ini(2);
I_error_1 = Con_ini(3);
difact = Con_ini(4);
Ad_1 = Con_ini(5);
Ad1_ = Con_ini(6);

umin = -100;
umax = 100;

Kp = -3.357670445385118;
Ki = 3.822951239710286;
Kd = 32.464560395668343;
N = 0.782109908780621;
Kpd = 0.285776886757601;
Kdp = 3.408050560944484;
N1 = 0.997168715666942;
Ka= 0.1; 

en =  Sp - Pv;
Ap = Kp*en;
Ad = Kd*(en-en_1) + N*Ad1_;
I_error = en + I_error_1 + Ka*difact;
Ai = Ki*I_error;
U1 = Ap + Ai + Ad;

Ap1 = Kpd * Pv;
Ad1 = Kdp * (Pv - yn_1) + N1*Ad_1;
U2 = Ap1 + Ad1;

Uc = U1 - U2;
us = Uc;


if Uc < umin 
    us = umin;
end
if Uc > umax 
    us = umax;
end

en_1 = en;
yn_1 = Pv;
I_error_1 = I_error;
difact = us - Uc;
Ad_1 = Ad1;
Ad1_ = Ad;
      
Con_out = [en_1; yn_1; I_error_1; difact; Ad_1; Ad1_];

== matlab function controladorContinua/Subsystem/2 DOF DISCRETA/MATLAB Function1 ==
  data: Sp input; us output; Pv input; Con_ini input; Con_out output
% function [us, Con_out] = fcn(Sp, Pv, Con_ini)
%  
% en_1 = Con_ini(1);
% u1_1 = Con_ini(2);
% Pv_1 = Con_ini(3);
% u2_1 = Con_ini(4);
% difact = Con_ini(5);
% umin = -100;
% umax = 100;
% kaw = 0.01; 
%  
% en = Sp - Pv;
% u1 = 0.153958966653420*en_1 + u1_1 + kaw*difact;
% u2 = 22.177058343736231*Pv - 21.573923642220816*(Pv_1) + 0.732201155629244*u2_1;
% un = u1-u2;
% us = un;
%  
% if un < umin 
%     us = umin;
% end
% if un > umax 
%     us = umax;
% end
%  
% en_1 = en;
% u1_1 = u1;
% Pv_1 = Pv;
% u2_1 = u2;
% difact = us - un;
%          
% Con_out = [en_1; u1_1; Pv_1;u2_1; difact];

function [us, Con_out] = fcn(Sp, Pv, Con_ini)

en_1 = Con_ini(1);
yn_1 = Con_ini(2);
I_error_1 = Con_ini(3);
difact = Con_ini(4);
Ad_1 = Con_ini(5);
Ad1_ = Con_ini(6);

umin = -100;
umax = 100;

Kp = -3.357670445385118;
Ki = 3.822951239710286;
Kd = 32.464560395668343;
N = 0.782109908780621;
Kpd = 0.285776886757601;
Kdp = 3.408050560944484;
N1 = 0.997168715666942;
Ka= 0.1; 

en =  Sp - Pv;
Ap = Kp*en;
Ad = Kd*(en-en_1) + N*Ad1_;
I_error = en + I_error_1 + Ka*difact;
Ai = Ki*I_error;
U1 = Ap + Ai + Ad;

Ap1 = Kpd * Pv;
Ad1 = Kdp * (Pv - yn_1) + N1*Ad_1;
U2 = Ap1 + Ad1;

Uc = U1 - U2;
us = Uc;


if Uc < umin 
    us = umin;
end
if Uc > umax 
    us = umax;
end

en_1 = en;
yn_1 = Pv;
I_error_1 = I_error;
difact = us - Uc;
Ad_1 = Ad1;
Ad1_ = Ad;
      
Con_out = [en_1; yn_1; I_error_1; difact; Ad_1; Ad1_];

== matlab function controladorContinua/Subsystem/2 DOF DISCRETA/Subsystem/MATLAB Function ==
  data: x input; PWM input; dx output; parametros input
function dx = fcn(x,PWM,parametros)

%ESTADOS
x1 = x(1);
x2 = x(2);
x3 = x(3);

%Parametros
R = parametros(1);
L = parametros(2);
Ki = parametros(3);
Kv = parametros(4);
Jm = parametros(5);
Jl = parametros(6);
Bm = parametros(7);
Bl = parametros(8);
n = parametros(9);
g = parametros(10);
d = parametros(11);
m = parametros(12);

%EXPRESIONES
% Jt = Jm*n^2 +Jl;
% f1 = (1/L)*(((7*PWM)/100) - R*x1 - Kv*x2*n);
% f2 = (1/Jt)*(Ki*x1*n - (Bm*n^2 + Bl)*x2 - m*g*d*sin(x3));
% f3 = x2;

% MODELO 2 ESTADOS I TL WL  SALIDA TL WL
f1 = (((7*PWM)/100)-Kv*x3*n-R*x1)/(L); %di/dt
f2 = x3; %d0l/dt = Wl
f3 = ((Ki*x1*n)-x3*(Bm*n^2+Bl)-(m*g*d*sin(x2)))/(Jl+Jm*n^2);  %dwl/dt 

dx = [f1; f2; f3];

== matlab function controladorContinua/CASCADA/MATLAB Function1 ==
  data: Sp input; u2 output; Pv input; Pv1 input; Con_ini input; Con_out output
function [u2,Con_out] = fcn(Sp,Pv,Pv1,Con_ini)

en_1 = Con_ini(1);
en_2 = Con_ini(2);
u1_1 = Con_ini(3);
u1_2 = Con_ini(4);
en2_1 = Con_ini(5);
en2_2 = Con_ini(6);
u2_1 = Con_ini(7);
u2_2 = Con_ini(8);

en = Sp - Pv;
u1 = 25.896804588396275*en -26.906839434709909*en_1 + 7.014080201415831*en_2 + 1.371242422443549*u1_1 - 0.371242422443549*u1_2;

en_2 = en_1;
en_1 = en;
u1_2 = u1_1;
u1_1 = u1;

en2 = u1 - Pv1;
u2 = 3.269366127619914*en2 -0.112980779954379*en2_1 + 1.106272350916589*en2_2 + 1.999700044995500*u2_1 - 0.999700044995500*u2_2;
en2_2 = en2_1;
en2_1 = en2;
u2_2 = u2_1;
u2_1 = u2;


Con_out = [en_1; en_2; u1_1; u1_2; en2_1; en2_2; u2_1; u2_2];

== matlab function controladorContinua/ESTADOS/Subsystem2/MATLAB Function ==
  data: x input; PWM input; dx output; parametros input
function dx = fcn(x,PWM,parametros)

%ESTADOS
x1 = x(1);
x2 = x(2);

%Parametros
R = parametros(1);
L = parametros(2);
Ki = parametros(3);
Kv = parametros(4);
Jm = parametros(5);
Jl = parametros(6);
Bm = parametros(7);
Bl = parametros(8);
n = parametros(9);
g = parametros(10);
d = parametros(11);
m = parametros(12);

%EXPRESIONES
f1 = x2; %d0l/dt = Wl
f2= ((Ki*(((7*PWM/100)-(Kv*x2*n)/R))*n)-x2*(Bm*n^2+Bl)-(m*g*d*sin(x1)))/(Jl+Jm*n^2);

dx = [f1; f2];
